simulink subsystem "BatteryMappedSSC"  (R2024a)
settings: Solver=VariableStepAuto  StartTime=0.0  StopTime=10.0  RelTol=1e-3
undefined symbols (not defined in the file): BattInfo, BattNeg, BattPos, BMSSensors, PlntBattChrgMax, PlntBattCp, PlntBattIntrnRes, PlntBattMass, PlntBattNumCellPar, PlntBattNumCellSer, PlntBattOpenCirctVolt
libraries: fl_lib x9, nesl_utility_internal x3, nesl_utility x2, batteryecm_lib x1
settings Model: ModifiedByFormat=The MathWorks, Inc.  Creator=The MathWorks, Inc.  LastModifiedBy=The MathWorks, Inc.
settings OptimizationCC: ReuseModelBlockBuffer=off
settings DebuggingCC: SubsystemReferenceDiagnosticForUnitTest=warning
settings RTWCC: GPUComputeCapability=3.5

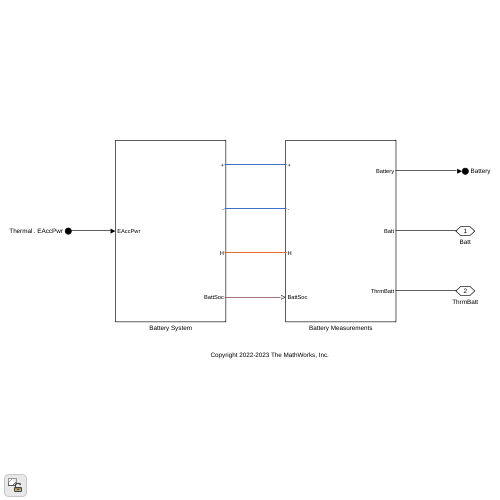
[thumbnail: Simulink's stored preview of the top-level diagram]
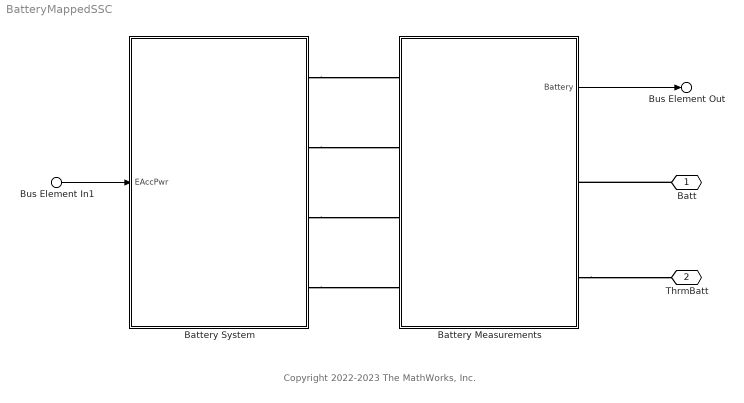
== system BatteryMappedSSC ==
  note: Copyright 2022-2023 The MathWorks, Inc.
  Bus Element In1 : Inport  PortName=Thermal  Element=EAccPwr
  Battery Measurements : Subsystem
  Battery System : Subsystem
  Batt : PMIOPort  Side=Right
  ThrmBatt : PMIOPort  Port=2  Side=Right
  Bus Element Out : Outport  PortName=Battery
  wires:
  Bus Element In1/1 -> Battery System/1(EAccPwr)
  Battery Measurements/1(Battery) -> Bus Element Out/1
  connections:
  Battery Measurements/RConn2 -- ThrmBatt/RConn1
  Batt/RConn1 -- Battery Measurements/RConn1
  Battery System/RConn4 -- Battery Measurements/LConn4
  Battery System/RConn3 -- Battery Measurements/LConn3
  Battery System/RConn2 -- Battery Measurements/LConn2
  Battery System/RConn1 -- Battery Measurements/LConn1

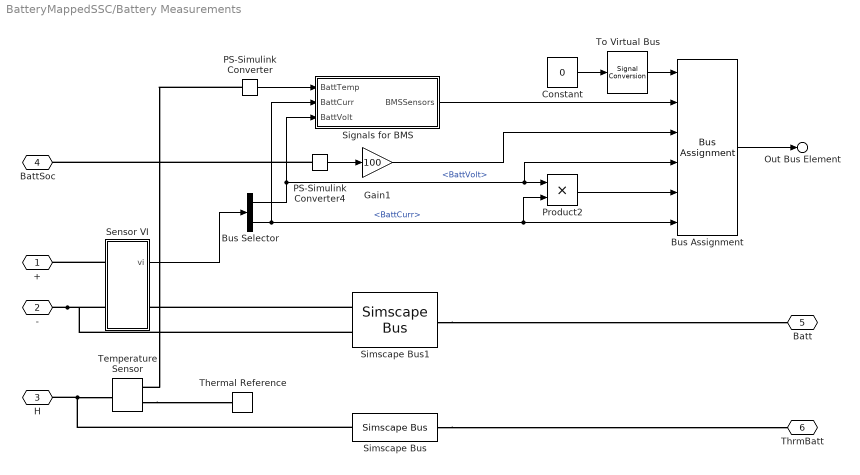
== system BatteryMappedSSC/Battery Measurements ==
  Bus Assignment : BusAssignment  AssignedSignals=BMSSensors,BattInfo.BattSoc,BattInfo.BattVolt,BattInfo.BattPwr,BattInfo.BattCurr
  Bus Selector : BusSelector  OutputSignals=BattVolt,BattCurr
  Constant : Constant  Value=0  OutDataTypeStr=Bus: BatteryBUS  SampleTime=Inf
  Gain1 : Gain  Gain=100
  PS-Simulink Converter : nesl_utility/PS-Simulink Converter  PhysicalDomain=network_engine_domain  SubClassName=ps_output  LeftPortType=input  RightPortType=output  PseudoPeriodic=off  Frequencies=[]  VectorFormat=inherit  Unit=inherit  AffineConversion=off
  PS-Simulink Converter4 : nesl_utility_internal/PS-Simulink Converter  PhysicalDomain=network_engine_domain  SubClassName=ps_output  LeftPortType=input  RightPortType=output  PseudoPeriodic=off  Frequencies=[]  VectorFormat=1-D array  Unit=1  AffineConversion=off
  Product2 : Product
  Sensor VI : Subsystem
  Signals for BMS : Subsystem
  Simscape Bus : SimscapeBus  HierarchyStrings=ThrmBatt1
  Simscape Bus1 : SimscapeBus  HierarchyStrings=BattPos;BattNeg
  Temperature Sensor : fl_lib/Thermal/Thermal Sensors/Temperature Sensor  temperature_measure=foundation.enum.MeasurementReference.difference
  Thermal Reference : fl_lib/Thermal/Thermal Elements/Thermal Reference
  To Virtual Bus : SignalConversion  ConversionOutput=Virtual bus  OverrideOpt=off
  + : PMIOPort  Side=Left
  - : PMIOPort  Port=2  Side=Left
  H : PMIOPort  Port=3  Side=Left
  BattSoc : PMIOPort  Port=4  Side=Left
  Batt : PMIOPort  Port=5  Side=Right
  ThrmBatt : PMIOPort  Port=6  Side=Right
  Out Bus Element : Outport  PortName=Battery
  wires:
  Sensor VI/1(vi) -> Bus Selector/1
  PS-Simulink Converter/1 -> Signals for BMS/1(BattTemp)
  Bus Selector/2 -> Signals for BMS/2(BattCurr), Bus Assignment/6, Product2/2  "<BattCurr>"
  Gain1/1 -> Bus Assignment/3
  Signals for BMS/1(BMSSensors) -> Bus Assignment/2
  PS-Simulink Converter4/1 -> Gain1/1
  Product2/1 -> Bus Assignment/5
  Bus Selector/1 -> Bus Assignment/4, Product2/1, Signals for BMS/3(BattVolt)  "<BattVolt>"
  Constant/1 -> To Virtual Bus/1
  Bus Assignment/1 -> Out Bus Element/1
  To Virtual Bus/1 -> Bus Assignment/1
  connections:
  Temperature Sensor/RConn1 -- Thermal Reference/LConn1
  PS-Simulink Converter/LConn1 -- Temperature Sensor/RConn2
  Sensor VI/LConn1 -- +/RConn1
  -/RConn1 -- Sensor VI/LConn2 -- Simscape Bus1/LConn2
  PS-Simulink Converter4/LConn1 -- BattSoc/RConn1
  Simscape Bus/LConn1 -- H/RConn1 -- Temperature Sensor/LConn1
  Simscape Bus/RConn1 -- ThrmBatt/RConn1
  Simscape Bus1/RConn1 -- Batt/RConn1
  Simscape Bus1/LConn1 -- Sensor VI/RConn1

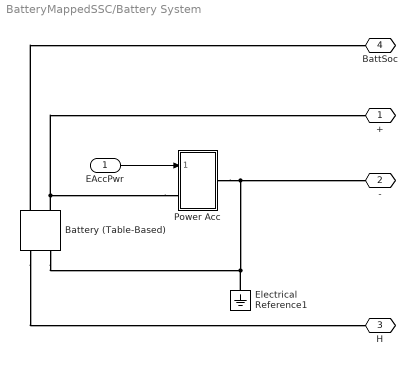
== system BatteryMappedSSC/Battery System ==
  EAccPwr : Inport
  Battery (Table-Based) : batteryecm_lib/Battery (Table-Based)  Tag={'toolbox/physmod/battery/shared_library/m/batteryecm_lib_parts';'Battery__Table_Based_/Molicel/INR_21700_P45B.xml'}  SOC_vec=PlntBattSocBpt  T_dependence=simscape.enum.tablebattery.temperature_dependence.yes  prm_dir=simscape.enum.tablebattery.prm_dir.noCurrentDirectionality  T_vec=PlntBattTempBpt degC  V0_mat=PlntBattOpenCirctVolt*PlntBattNumCellSer V  V0_vec=[3.17242 3.18272 3.19302 3.20331 3.21361 3.22391 3.23421 3.24451 3.25481 3.2651 3.2754 3.2857 3.296 3.3063 3.31659 3.32689 3.33719 3.34749 3.35779 3.36809 3.37838 3.38868 3.39898 3.40928 3.41958 3.42988 3.44017 3.45047 3.46077 3.47107 3.48137 3.49166 3.50196 3.51226 3.52256 3.53286 3.54316 3.55345 3.56375 3.57405 3.58435 3.59465 3.60495 3.61524 3.62554 3.63584 3.64614 3.65644 3.66673 3.67703 3.68733 3.69763 3.71041 3.72113 3.72997 3.73882 3.74912 3.75936 3.76951 3.7791 3.78865 3.79787 3.80709 3.8161 3.82509 3.83409 3.84308 3.85207 3.86107 3.87006 3.87901 3.88831 3.89824 3.90887 3.91951 3.93012 3.94073 3.95138 3.96184 3.97226 3.98268 3.99311 4.0032 4.01221 4.01944 4.02668 4.03286 4.03874 4.04383 4.0488 4.05377 4.05873 4.06312 4.06753 4.07333 4.08117 4.08904 4.09911 4.11111 4.13802 4.16831] V  V_range=[2.25 Inf]*PlntBattNumCellSer V  R0_mat=PlntBattIntrnRes*(PlntBattNumCellSer/PlntBattNumCellPar) Ohm  R0_vec=[0.02095 0.01921 0.01774 0.0166 0.01557 0.01469 0.01398 0.01338 0.01283 0.01239 0.01196 0.01155 0.01116 0.01079 0.01042 0.01007 0.00974 0.00949 0.00924 0.009 0.00876 0.00855 0.00843 0.00832 0.00826 0.00825 0.00825 0.00826 0.00827 0.00828 0.0083 0.00834 0.00838 0.00842 0.00848 0.00855 0.00863 0.00871 0.00879 0.00887 0.00895 0.00903 0.00911 0.00918 0.00925 0.00931 0.00938 0.00946 0.00953 0.00961 0.00968 0.00976 0.00991 0.01 0.01003 0.01006 0.01013 0.01022 0.0103 0.01037 0.01043 0.01049 0.01055 0.01061 0.01066 0.01072 0.01077 0.01082 0.01088 0.01093 0.01099 0.01105 0.01114 0.01125 0.01136 0.01148 0.01161 0.01175 0.01188 0.01202 0.01215 0.01228 0.01241 0.01253 0.01261 0.01269 0.01275 0.0128 0.01285 0.01289 0.01294 0.01298 0.01296 0.01292 0.01292 0.01288 0.01282 0.0128 0.01232 0.01214 0.00952] Ohm  R0_dis_mat=[.0117, .0085, .009; .011, .0085, .009; .0114, .0087, .0092; .0107, .0082, .0088; .0107, .0083, .0091; .0113, .0085, .0089; .0116, .0085, .0089] % Parameter not set Ohm  R0_dis_vec=[.0085, .0085, .0087, .0082, .0083, .0085, .0085] % Parameter not set Ohm  R0_ch_mat=[.0117, .0085, .009; .011, .0085, .009; .0114, .0087, .0092; .0107, .0082, .0088; .0107, .0083, .0091; .0113, .0085, .0089; .0116, .0085, .0089] % Parameter not set Ohm  R0_ch_vec=[.0085, .0085, .0087, .0082, .0083, .0085, .0085] % Parameter not set Ohm  AH=PlntBattChrgMax*PlntBattNumCellPar hr*A  prm_leak=simscape.enum.tablebattery.prm_leak.disabled  Rleak_vec=[8000, 7000, 6000] % Parameter not set Ohm  Rleak=7e3 % Parameter not set Ohm  extrapolation_option=simscape.enum.extrapolation.nearest  SOC_port=simscape.enum.tablebattery.enable.yes  prm_dyn=simscape.enum.tablebattery.prm_dyn.off  R1_mat=[.0109, .0029, .0013; .0069, .0024, .0012; .0047, .0026, .0013; .0034, .0016, .001; .0033, .0023, .0014; .0033, .0018, .0011; .0028, .0017, .0011] % Parameter not set Ohm  R1_vec=[.0029, .0024, .0026, .0016, .0023, .0018, .0017] % Parameter not set Ohm  tau1_mat=[20, 36, 39; 31, 45, 39; 109, 105, 61; 36, 29, 26; 59, 77, 67; 40, 33, 29; 25, 39, 33] % Parameter not set s  tau1_vec=[36, 45, 105, 29, 77, 33, 39] % Parameter not set s  R2_mat=[.0109, .0029, .0013; .0069, .0024, .0012; .0047, .0026, .0013; .0034, .0016, .001; .0033, .0023, .0014; .0033, .0018, .0011; .0028, .0017, .0011] % Parameter not set Ohm  R2_vec=[.0029, .0024, .0026, .0016, .0023, .0018, .0017] % Parameter not set Ohm  tau2_mat=[20, 36, 39; 31, 45, 39; 109, 105, 61; 36, 29, 26; 59, 77, 67; 40, 33, 29; 25, 39, 33] % Parameter not set s  tau2_vec=[36, 45, 105, 29, 77, 33, 39] % Parameter not set s  R3_mat=[.0109, .0029, .0013; .0069, .0024, .0012; .0047, .0026, .0013; .0034, .0016, .001; .0033, .0023, .0014; .0033, .0018, .0011; .0028, .0017, .0011] % Parameter not set Ohm  R3_vec=[.0029, .0024, .0026, .0016, .0023, .0018, .0017] % Parameter not set Ohm  tau3_mat=[20, 36, 39; 31, 45, 39; 109, 105, 61; 36, 29, 26; 59, 77, 67; 40, 33, 29; 25, 39, 33] % Parameter not set s  tau3_vec=[36, 45, 105, 29, 77, 33, 39] % Parameter not set s  R4_mat=[.0109, .0029, .0013; .0069, .0024, .0012; .0047, .0026, .0013; .0034, .0016, .001; .0033, .0023, .0014; .0033, .0018, .0011; .0028, .0017, .0011] % Parameter not set Ohm  R4_vec=[.0029, .0024, .0026, .0016, .0023, .0018, .0017] % Parameter not set Ohm  tau4_mat=[20, 36, 39; 31, 45, 39; 109, 105, 61; 36, 29, 26; 59, 77, 67; 40, 33, 29; 25, 39, 33] % Parameter not set s  tau4_vec=[36, 45, 105, 29, 77, 33, 39] % Parameter not set s  R5_mat=[.0109, .0029, .0013; .0069, .0024, .0012; .0047, .0026, .0013; .0034, .0016, .001; .0033, .0023, .0014; .0033, .0018, .0011; .0028, .0017, .0011] % Parameter not set Ohm  R5_vec=[.0029, .0024, .0026, .0016, .0023, .0018, .0017] % Parameter not set Ohm  tau5_mat=[20, 36, 39; 31, 45, 39; 109, 105, 61; 36, 29, 26; 59, 77, 67; 40, 33, 29; 25, 39, 33] % Parameter not set s  tau5_vec=[36, 45, 105, 29, 77, 33, 39] % Parameter not set s  prm_fade=simscape.enum.tablebattery.prm_fade.tableN  N0=100 % Parameter not set  dV0=0 % Parameter not set  dR0=0 % Parameter not set  dAH=0 % Parameter not set  dRleak=0 % Parameter not set  dR1=0 % Parameter not set  dR2=0 % Parameter not set  dR3=0 % Parameter not set  dR4=0 % Parameter not set  dR5=0 % Parameter not set  N0vec=[0 6 11 16 21 26 31 36 41 46 51 56 61 66 71 76 81 86 91 96 101 106 111 116 121 126 131 136 141 146 151 156 161 166 171 176 181 186 191 196 201 206 211 216 221 226 231 236 241 246 251 256 261 266 271 276 281 286 291 296 301 306 311 316 321 326 331 336 341 346 351 356 361 366 371 376 381 386 391 396 401 406 411 416 421 426 431 436 441 446 451 456 461 466 471 476 481 486 491 496]  Tfadevec=[298.15, 323.15] % Parameter not set K  dV0vec=[0 -0.0674 -0.1349 -0.2023 -0.2697 -0.3371 -0.4046 -0.472 -0.5394 -0.6069 -0.6828 -0.7561 -0.8245 -0.8929 -0.9613 -1.0297 -1.0981 -1.1664 -1.2348 -1.3032 -1.3773 -1.4186 -1.4598 -1.5011 -1.5424 -1.5836 -1.6249 -1.6652 -1.6999 -1.7345 -1.7691 -1.8038 -1.8384 -1.8731 -1.908 -1.9398 -1.9715 -2.0033 -2.0351 -2.0669 -2.0986 -2.1303 -2.162 -2.1976 -2.2332 -2.2687 -2.2977 -2.3239 -2.3502 -2.3765 -2.4028 -2.4264 -2.4464 -2.4663 -2.4863 -2.5063 -2.5263 -2.5462 -2.5661 -2.5849 -2.6031 -2.6212 -2.6407 -2.6612 -2.6817 -2.7022 -2.7227 -2.7432 -2.7637 -2.7842 -2.8047 -2.8253 -2.8458 -2.8662 -2.8858 -2.9054 -2.9249 -2.9445 -2.9641 -2.9837 -3.0037 -3.0238 -3.0439 -3.064 -3.0841 -3.1042 -3.1267 -3.1499 -3.1731 -3.1989 -3.2248 -3.2508 -3.2781 -3.3053 -3.3326 -3.3598 -3.387 -3.4171 -3.449 -3.4809]  dR0vec=[0 0 0 0 0 0 0 0 0 0 0 0 0 0 0 0 0 0 0 0 0 0 0 0 0 0 0 0 0 0 0 0 0 0 0 0 0 0 0 0 0 0 0 0 0 0 0 0 0 0 0 0 0 0 0 0 0 0 0 0 0 0 0 0 0 0 0 0 0 0 0 0 0 0 0 0 0 0 0 0 0 0 0 0 0 0 0 0 0 0 0 0 0 0 0 0 0 0 0 0] % Parameter assumed  dAHvec=[0 -0.093 -0.186 -0.278 -0.371 -0.464 -0.557 -0.649 -0.742 -0.835 -0.94 -1.045 -1.151 -1.257 -1.363 -1.469 -1.575 -1.681 -1.787 -1.893 -2.017 -2.161 -2.304 -2.447 -2.591 -2.734 -2.877 -3.021 -3.164 -3.307 -3.451 -3.594 -3.737 -3.881 -4.032 -4.201 -4.369 -4.538 -4.706 -4.874 -5.043 -5.211 -5.38 -5.569 -5.758 -5.947 -6.135 -6.324 -6.513 -6.702 -6.891 -7.08 -7.269 -7.458 -7.647 -7.836 -8.025 -8.214 -8.403 -8.582 -8.754 -8.927 -9.099 -9.271 -9.443 -9.615 -9.787 -9.96 -10.132 -10.304 -10.476 -10.648 -10.82 -10.992 -11.156 -11.32 -11.485 -11.649 -11.814 -11.978 -12.143 -12.307 -12.471 -12.636 -12.8 -12.965 -13.129 -13.293 -13.458 -13.641 -13.825 -14.008 -14.192 -14.376 -14.56 -14.743 -14.927 -15.111 -15.295 -15.478]  dRleakvec=[0, 0, 0, 0] % Parameter not set  dR1vec=[0, 0, 0, 0] % Parameter not set  dR2vec=[0, 0, 0, 0] % Parameter not set  dR3vec=[0, 0, 0, 0] % Parameter not set  dR4vec=[0, 0, 0, 0] % Parameter not set  dR5vec=[0, 0, 0, 0] % Parameter not set  dV0mat=[0, 0; 0, 0; 0, 0; 0, 0] % Parameter not set  dR0mat=[0, 0; 0, 0; 0, 0; 0, 0] % Parameter not set  dAHmat=[0, 0; 0, 0; 0, 0; 0, 0] % Parameter not set  dRleakmat=[0, 0; 0, 0; 0, 0; 0, 0] % Parameter not set  dR1mat=[0, 0; 0, 0; 0, 0; 0, 0] % Parameter not set  dR2mat=[0, 0; 0, 0; 0, 0; 0, 0] % Parameter not set  dR3mat=[0, 0; 0, 0; 0, 0; 0, 0] % Parameter not set  dR4mat=[0, 0; 0, 0; 0, 0; 0, 0] % Parameter not set  dR5mat=[0, 0; 0, 0; 0, 0; 0, 0] % Parameter not set  prm_age_modeling=simscape.enum.tablebattery.prm_age_modeling.equation  storage_dt_age_vec=[0] % Parameter not set d  storage_T_age_vec=[273] % Parameter not set K  prm_age_OCV=simscape.enum.tablebattery.prm_age_OCV.OCV  OCV_age=0.9 % Parameter not set  SOC_age=0.6 % Parameter not set  prm_age_resistance=simscape.enum.tablebattery.prm_age.disabled  OCV_scaling_age_resistance=2.2134e6 % Parameter not set  OCV_offset_age_resistance=1.632e6 % Parameter not set  temp_exp_age_resistance=0.515833569 % Parameter not set V  t_exp_age_resistance=0.75 % Parameter not set  T_age_vec_resistance=[273.15, 298.15, 323.15] % Parameter not set K  dt_age_vec_resistance=[0, 90, 180, 270] % Parameter not set d  dR0_age_vec=[0, 0, 0] % Parameter not set  t_meas_dR0_age=100 % Parameter not set d  dR0_age_mat=[0, 0, 0; 0, 0, 0; 0, 0, 0; 0, 0, 0] % Parameter not set  prm_age_capacity=simscape.enum.tablebattery.prm_age.disabled  OCV_scaling_age_capacity=1.5097e07 % Parameter not set  OCV_offset_age_capacity=8.3625e06 % Parameter not set  temp_exp_age_capacity=0.6011 % Parameter not set V  t_exp_age_capacity=0.75 % Parameter not set  T_age_vec_capacity=[273.15, 298.15, 323.15] % Parameter not set K  dt_age_vec_capacity=[0, 90, 180, 270] % Parameter not set d  dAH_age_vec=[0, 0, 0] % Parameter not set  t_meas_dAH_age=100 % Parameter not set d  dAH_age_mat=[0, 0, 0; 0, 0, 0; 0, 0, 0; 0, 0, 0] % Parameter not set  thermal_port=simscape.enum.thermaleffects.model  temperature=298.15 % Parameter not set K  thermal_mass=PlntBattMass*PlntBattCp J/K  i_specify=off  i_priority=None  i=0 A  i_nominal_specify=off  i_nominal_value=1  i_nominal_unit=A  v_specify=off  v_priority=None  v=0 V  v_nominal_specify=off  v_nominal_value=1  v_nominal_unit=V  stateOfCharge_specify=on  stateOfCharge_priority=High  stateOfCharge=PlntBattSocInit  stateOfCharge_nominal_specify=off  stateOfCharge_nominal_value=1  stateOfCharge_nominal_unit=1  num_cycles_specify=off  num_cycles_priority=High  num_cycles=0  num_cycles_nominal_specify=off  num_cycles_nominal_value=1  num_cycles_nominal_unit=1  cell_temperature_specify=on  cell_temperature_priority=High  cell_temperature=EnvAirTemp K  cell_temperature_nominal_specify=off  cell_temperature_nominal_value=1  cell_temperature_nominal_unit=K
      settings: AttributesFormatString=Molicel:INR_21700_P45B
  Electrical Reference1 : fl_lib/Electrical/Electrical Elements/Electrical Reference
  Power Acc : Subsystem
  + : PMIOPort  Side=Right
  - : PMIOPort  Port=2  Side=Right
  H : PMIOPort  Port=3  Side=Right
  BattSoc : PMIOPort  Port=4  Side=Right
  wires:
  EAccPwr/1 -> Power Acc/1(P_Acc)
  connections:
  Battery (Table-Based)/RConn2 -- H/RConn1
  Power Acc/LConn1 -- Battery (Table-Based)/LConn1 -- +/RConn1
  Electrical Reference1/LConn1 -- Battery (Table-Based)/RConn1 -- Power Acc/RConn1 -- -/RConn1
  Battery (Table-Based)/LConn2 -- BattSoc/RConn1

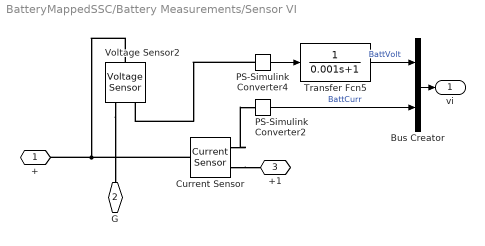
== system BatteryMappedSSC/Battery Measurements/Sensor VI ==
  Bus Creator : BusCreator  Inputs=2
  Current Sensor : fl_lib/Electrical/Electrical Sensors/Current Sensor
  PS-Simulink Converter2 : nesl_utility_internal/PS-Simulink Converter  PhysicalDomain=network_engine_domain  SubClassName=ps_output  LeftPortType=input  RightPortType=output  PseudoPeriodic=off  Frequencies=[]  VectorFormat=1-D array  Unit=1  AffineConversion=off
  PS-Simulink Converter4 : nesl_utility_internal/PS-Simulink Converter  PhysicalDomain=network_engine_domain  SubClassName=ps_output  LeftPortType=input  RightPortType=output  PseudoPeriodic=off  Frequencies=[]  VectorFormat=1-D array  Unit=1  AffineConversion=off
  Transfer Fcn5 : TransferFcn  Denominator=[0.001 1]
  Voltage Sensor2 : fl_lib/Electrical/Electrical Sensors/Voltage Sensor
  + : PMIOPort  Side=Left
  G : PMIOPort  Port=2  Side=Left
  +1 : PMIOPort  Port=3  Side=Right
  vi : Outport
  wires:
  Bus Creator/1 -> vi/1
  PS-Simulink Converter4/1 -> Transfer Fcn5/1
  PS-Simulink Converter2/1 -> Bus Creator/2  "BattCurr"
  Transfer Fcn5/1 -> Bus Creator/1  "BattVolt"
  connections:
  Current Sensor/RConn1 -- PS-Simulink Converter2/LConn1
  Voltage Sensor2/RConn2 -- G/RConn1
  Current Sensor/RConn2 -- +1/RConn1
  PS-Simulink Converter4/LConn1 -- Voltage Sensor2/RConn1
  Voltage Sensor2/LConn1 -- Current Sensor/LConn1 -- +/RConn1

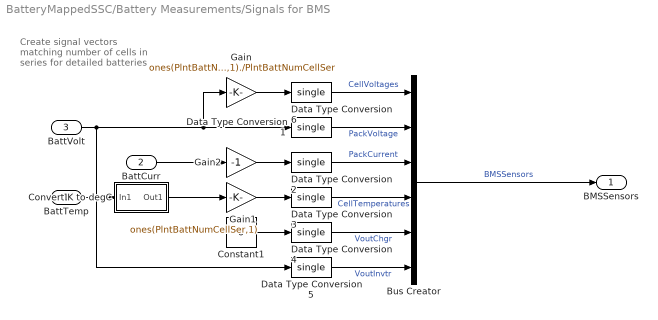
== system BatteryMappedSSC/Battery Measurements/Signals for BMS ==
  note: Create signal vectors
      | matching number of
      | cells in series for
      | detailed batteries
  BattTemp : Inport
  BattCurr : Inport  Port=2
  BattVolt : Inport  Port=3
  Bus Creator : BusCreator  Inputs=6
  Constant1 : Constant  Value=0  SampleTime=-1
  Convert K to degC : Subsystem
  Data Type Conversion{1..6} (6 alike) : DataTypeConversion  OutDataTypeStr=single  SaturateOnIntegerOverflow=off  RndMeth=Floor
  Gain : Gain  Gain=ones(PlntBattNumCellSer,1)./PlntBattNumCellSer
  Gain1 : Gain  Gain=ones(PlntBattNumCellSer,1)
  Gain2 : Gain  Gain=-1
  BMSSensors : Outport
  wires:
  Bus Creator/1 -> BMSSensors/1  "BMSSensors"
  Data Type Conversion3/1 -> Bus Creator/4  "CellTemperatures"
  Data Type Conversion2/1 -> Bus Creator/3  "PackCurrent"
  Data Type Conversion6/1 -> Bus Creator/1  "CellVoltages"
  Data Type Conversion1/1 -> Bus Creator/2  "PackVoltage"
  Convert K to degC/1(Out1) -> Gain1/1
  Gain2/1 -> Data Type Conversion2/1
  Data Type Conversion5/1 -> Bus Creator/6  "VoutInvtr"
  Gain1/1 -> Data Type Conversion3/1
  Data Type Conversion4/1 -> Bus Creator/5  "VoutChgr"
  BattTemp/1 -> Convert K to degC/1(In1)
  Gain/1 -> Data Type Conversion6/1
  BattVolt/1 -> Data Type Conversion5/1, Gain/1, Data Type Conversion1/1
  Constant1/1 -> Data Type Conversion4/1
  BattCurr/1 -> Gain2/1

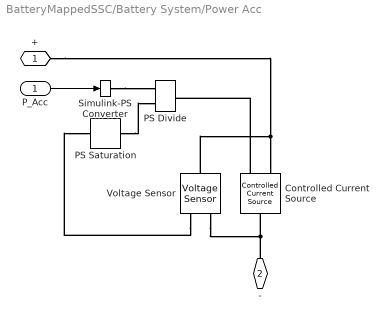
== system BatteryMappedSSC/Battery System/Power Acc ==
  P_Acc : Inport
  Controlled Current Source : fl_lib/Electrical/Electrical Sources/Controlled Current Source
  PS Divide : fl_lib/Physical Signals/Functions/PS Divide
  PS Saturation : fl_lib/Physical Signals/Nonlinear Operators/PS Saturation  upper_limit=Inf V  lower_limit=min(PlntBattOpenCirctVolt, [], 'all')*PlntBattNumCellSer V
  Simulink-PS Converter : nesl_utility/Simulink-PS Converter  PhysicalDomain=network_engine_domain  SubClassName=ps_input  LeftPortType=input  RightPortType=output  PseudoPeriodic=off  Frequencies=[]  NoiseDistribution=none  NoiseParameters=[]  Unit=W  AffineConversion=off  FilteringAndDerivatives=provide  SimscapeFilterOrder=1  InputFilterTimeConstant=0.001  UdotUserProvided=0
  Voltage Sensor : fl_lib/Electrical/Electrical Sensors/Voltage Sensor
  + : PMIOPort  Side=Left
  - : PMIOPort  Port=2  Side=Right
  wires:
  P_Acc/1 -> Simulink-PS Converter/1
  connections:
  Controlled Current Source/RConn1 -- PS Divide/RConn1
  +/RConn1 -- Voltage Sensor/LConn1 -- Controlled Current Source/RConn2
  Voltage Sensor/RConn2 -- -/RConn1 -- Controlled Current Source/LConn1
  Simulink-PS Converter/RConn1 -- PS Divide/LConn1
  Voltage Sensor/RConn1 -- PS Saturation/LConn1
  PS Saturation/RConn1 -- PS Divide/LConn2

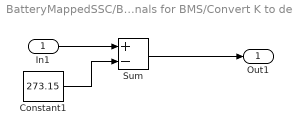
== system BatteryMappedSSC/Battery Measurements/Signals for BMS/Convert K to degC ==
  In1 : Inport
  Constant1 : Constant  Value=273.15
  Sum : Sum  Inputs=+-
  Out1 : Outport
  wires:
  In1/1 -> Sum/1
  Constant1/1 -> Sum/2
  Sum/1 -> Out1/1
